simulink model "DDPGImpedance"  (R2024b)
settings: Solver=ode4  StartTime=0.001  StopTime=28  FixedStep=1e-4  RelTol=1e-3
libraries: simulink x2, slpidlib x1, rllib x1
settings Model: PacingRate=2  Creator=edwar  LastModifiedBy=edwar

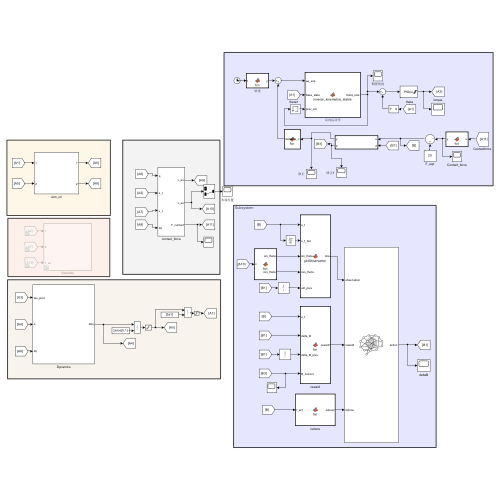
[thumbnail: Simulink's stored preview of the top-level diagram]
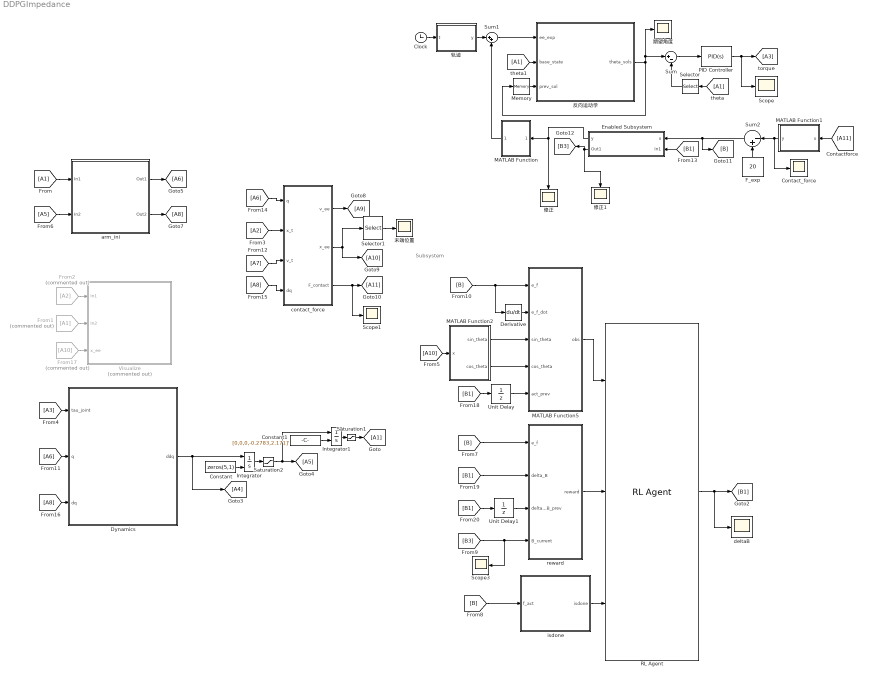
== system DDPGImpedance ==
  note: Subsystem
  Clock : Clock
  Constant : Constant  Value=zeros(5,1)
  Constant1 : Constant  Value=[0,0,0,-0.2783,2.171]'
  Contact_force : Scope
  Derivative : Derivative
  Dynamics : Subsystem
  Enabled Subsystem : Subsystem  TreatAsAtomicUnit=on
  F_exp : Constant  Value=20
  From1 : From  Commented=on  GotoTag=A1
  From17 : From  Commented=on  GotoTag=A10
  From2 : From  Commented=on  GotoTag=A2
  Integrator : Integrator  InitialConditionSource=external  InitialCondition=[0,0,0,0,0]'
  Integrator1 : Integrator  InitialConditionSource=external  InitialCondition=zeros(5,1)
  MATLAB Function : MATLAB Function  TreatAsAtomicUnit=on
  MATLAB Function1 : MATLAB Function  TreatAsAtomicUnit=on
  MATLAB Function2 : MATLAB Function  TreatAsAtomicUnit=on
  MATLAB Function5 : MATLAB Function  TreatAsAtomicUnit=on
  Memory : Memory  InitialCondition=[0;0]  InheritSampleTime=on
  PID Controller : slpidlib/PID Controller  Controller=PID  Form=Parallel  TimeDomain=Continuous-time  UseExternalTs=off  SampleTime=-1  IntegratorMethod=Forward Euler  FilterMethod=Forward Euler  ControllerParametersSource=internal  P=0.5  I=0  UseKiTs=off  D=0.8  UseExternalDerivativeSource=off  N=100  UseFilter=on  TunerSelectOption=Transfer Function Based (PID Tuner App)  InitialConditionSource=internal  InitialConditionForIntegrator=0  InitialConditionForFilter=0  DifferentiatorICPrevScaledInput=0  ExternalReset=none  TrackingMode=off  Kt=1  LimitOutput=on  SatLimitsSource=internal  UpperSaturationLimit=1.4  LowerSaturationLimit=-1.4  LinearizeAsGain=on  AntiWindupMode=none  Kb=1  LimitIntegrator=off  UpperIntegratorSaturationLimit=inf  LowerIntegratorSaturationLimit=-inf  POutMin=[]  POutMax=[]  IOutMin=[]  IOutMax=[]  DOutMin=[]  DOutMax=[]  NOutMin=[]  NOutMax=[]  SumOutMin=[]  SumOutMax=[]  SaturationOutMin=[]  SaturationOutMax=[]  PParamMin=[]  PParamMax=[]  IParamMin=[]  IParamMax=[]  DParamMin=[]  DParamMax=[]  NParamMin=[]  NParamMax=[]  KbParamMin=[]  KbParamMax=[]  KtParamMin=[]  KtParamMax=[]  KbOutMin=[]  KbOutMax=[]  KtOutMin=[]  KtOutMax=[]  IntegratorOutMin=[]  IntegratorOutMax=[]  FilterOutMin=[]  FilterOutMax=[]  SumI1OutMin=[]  SumI1OutMax=[]  SumI2OutMin=[]  SumI2OutMax=[]  SumI3OutMin=[]  SumI3OutMax=[]  SumI4OutMin=[]  SumI4OutMax=[]  SumDOutMin=[]  SumDOutMax=[]  DifferentiatorOutMin=[]  DifferentiatorOutMax=[]  FilterDiffOutCoefMin=[]  FilterDiffOutCoefMax=[]  ReciprocalOutMin=[]  ReciprocalOutMax=[]  SumDenOutMin=[]  SumDenOutMax=[]  SumNumOutMin=[]  SumNumOutMax=[]  DivideOutMin=[]  DivideOutMax=[]  UdiffTsProdOutMin=[]  UdiffTsProdOutMax=[]  NTsProdOutMin=[]  NTsProdOutMax=[]  UintegralTsProdOutMin=[]  UintegralTsProdOutMax=[]  UngainTsProdOutMin=[]  UngainTsProdOutMax=[]  ClampingZeroOutDataTypeStr=Inherit: Inherit via back propagation  ClampingZeroOutMin=[]  ClampingZeroOutMax=[]  FilterDenConstantOutDataTypeStr=Inherit: Inherit via back propagation  FilterDenConstantOutMin=[]  FilterDenConstantOutMax=[]  PCopyOutDataTypeStr=Inherit: Inherit via back propagation  PCopyOutMin=[]  PCopyOutMax=[]  NCopyOutDataTypeStr=Inherit: Inherit via back propagation  NCopyOutMin=[]  NCopyOutMax=[]  IntegratorContinuousStateAttributes=''  IntegratorStateMustResolveToSignalObject=off  IntegratorRTWStateStorageClass=Auto  FilterContinuousStateAttributes=''  FilterStateMustResolveToSignalObject=off  FilterRTWStateStorageClass=Auto  ParallelPVariant=InternalParameters  IdealPVariant=Disabled  IVariant=InternalParameters  DVariant=InternalParameters  IntegratorVariant=Continuous  SatVariant=Enabled  AWVariant=Passthrough  PCopyVariant=Disabled  TRVariant=Disabled  FdbkBlocksVariant=Forward  IdealPFdbkVariant=Disabled  SatFdbkVariant=Disabled  DerivativeFilterVariant=ContFilter  NVariant=InternalParameters  NCopyVariant=Disabled  FilterICVariant=InternalICsFilter  IntegratorICVariant=InternalICs  ExternalResetVariant=Disabled  TRSumVariant=Passthrough  SumFdbkVariant=Disabled  SumVariant=Sum_PID  TsampFilterVariant=InternalTs  TsampNgainVariant=Passthrough  TsampIntegralVariant=Disabled_SignalSpec  ExternalSaturationOutDataTypeStr=Inherit: Same as second input  DerivativeSourceVariant=ErrorSignal  PreIntVariant=InternalPreInt
  RL Agent : rllib/RL Agent  Agent=agent  ExternalActionAsInput=off  ProvideLastAction=off  ProvideCumRwd=off  TreatAsDirectFeedthrough=on  UseStrictObservationDataTypes=off
  Saturation1 : Saturate  UpperLimit=[1.5,1.5,5*pi,2.5,2.5]'  LowerLimit=[-1.5,-1.5,-5*pi,-2.5,-2.5]'
  Saturation2 : Saturate  UpperLimit=[0.075,0.075,pi/6,4.2,4.2]'  LowerLimit=[-0.075,-0.075,-pi/6,-4.2,-4.2]'
  Scope : Scope
  Scope1 : Scope
  Scope3 : Scope
  Selector : Selector  InputPortWidth=5  IndexOptions=Index vector (dialog)  Indices=[4 5]  OutputSizes=1
  Selector1 : Selector  InputPortWidth=2  IndexOptions=Index vector (dialog)  Indices=[2]  OutputSizes=1
  Sum : Sum  Inputs=|+-
  Sum1 : Sum  Inputs=|++
  Sum2 : Sum  Inputs=|-+
  Unit Delay : UnitDelay  SampleTime=-1  HasFrameUpgradeWarning=on
  Unit Delay1 : UnitDelay  SampleTime=-1  HasFrameUpgradeWarning=on
  Visualize : Subsystem  Commented=on
  arm_ini : Subsystem
  contact_force : Subsystem
  deltaB : Scope
  isdone : MATLAB Function  TreatAsAtomicUnit=on
  reward : MATLAB Function  TreatAsAtomicUnit=on
  修正 : Scope
  修正1 : Scope
  反向运动学 : MATLAB Function  TreatAsAtomicUnit=on
  期望角度 : Scope
  末端位置 : Scope
  轨迹 : MATLAB Function  TreatAsAtomicUnit=on
  wires:
  Enabled Subsystem/1(y) -> 修正/1, MATLAB Function/1(delta_n)
  Integrator/1 -> Saturation2/1
  contact_force/1(v_ee) -> [A9]
  Dynamics/1(ddq) -> [A4], Integrator/1
  Sum1/1 -> 反向运动学/1(ee_exp)
  Sum/1 -> PID Controller/1
  [A7] -> contact_force/3(v_t)
  [A8] -> Dynamics/3(dq)
  [A5] -> arm_ini/2(In2)
  Memory/1 -> 反向运动学/3(prev_sol)
  MATLAB Function/1(dxdy) -> Sum1/2
  arm_ini/2(Out2) -> [A8]
  [A1] -> 反向运动学/2(base_state)
  From2/1 -> Visualize/1(In1)
  [A6] -> contact_force/1(q)
  轨迹/1(y) -> Sum1/1
  Saturation2/1 -> Integrator1/1, [A5]
  MATLAB Function1/1(y) -> Sum2/1, Contact_force/1
  [A1] -> arm_ini/1(In1)
  contact_force/2(x_ee) -> Selector1/1, [A10]
  PID Controller/1 -> Scope/1, [A3]
  [A2] -> contact_force/2(x_t)
  From1/1 -> Visualize/2(In2)
  Constant1/1 -> Integrator1/2
  Selector/1 -> Sum/2
  Constant/1 -> Integrator/2
  [A11] -> MATLAB Function1/1(u)
  反向运动学/1(theta_sols) -> 期望角度/1, Sum/1, Memory/1
  [A6] -> Dynamics/2(q)
  F_exp/1 -> Sum2/2
  [A1] -> Selector/1
  Integrator1/1 -> Saturation1/1
  Saturation1/1 -> [A1]
  Clock/1 -> 轨迹/1(t)
  [A3] -> Dynamics/1(tau_joint)
  arm_ini/1(Out1) -> [A6]
  [A8] -> contact_force/4(dq)
  contact_force/3(F_contact) -> Scope1/1, [A11]
  Sum2/1 -> Enabled Subsystem/1(u), [B]
  [B1] -> Enabled Subsystem/2(In1)
  Enabled Subsystem/2(Out1) -> 修正1/1, [B3]
  From17/1 -> Visualize/3(x_ee)
  [B1] -> Unit Delay/1
  [B1] -> Unit Delay1/1
  [B1] -> reward/2(delta_B)
  MATLAB Function2/2(cos_theta) -> MATLAB Function5/4(cos_theta)
  Unit Delay1/1 -> reward/3(delta_B_prev)
  reward/1(reward) -> RL Agent/2
  isdone/1(isdone) -> RL Agent/3
  [B] -> reward/1(e_f)
  MATLAB Function5/1(obs) -> RL Agent/1
  [B3] -> reward/4(B_current), Scope3/1
  Derivative/1 -> MATLAB Function5/2(e_f_dot)
  [B] -> isdone/1(f_act)
  Unit Delay/1 -> MATLAB Function5/5(act_prev)
  [A10] -> MATLAB Function2/1(x)
  RL Agent/1 -> [B1], deltaB/1
  MATLAB Function2/1(sin_theta) -> MATLAB Function5/3(sin_theta)
  [B] -> MATLAB Function5/1(e_f), Derivative/1
  Selector1/1 -> 末端位置/1

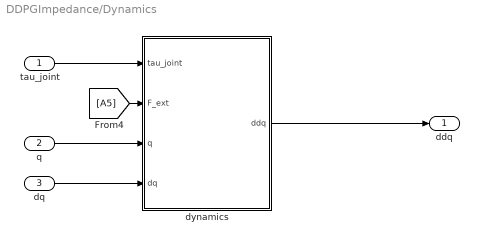
== system DDPGImpedance/Dynamics ==
  tau_joint : Inport
  q : Inport  Port=2
  dq : Inport  Port=3
  dynamics : MATLAB Function  TreatAsAtomicUnit=on
  ddq : Outport
  wires:
  tau_joint/1 -> dynamics/1(tau_joint)
  [A5] -> dynamics/2(F_ext)
  dq/1 -> dynamics/4(dq)
  dynamics/1(ddq) -> ddq/1
  q/1 -> dynamics/3(q)

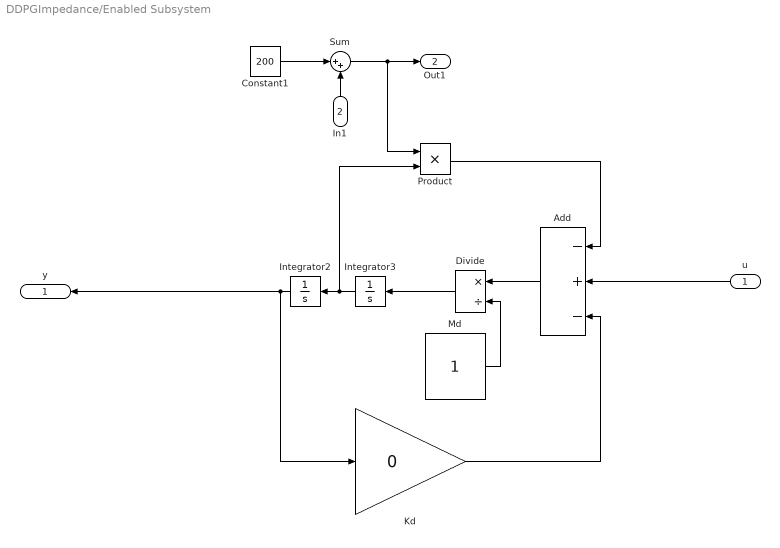
== system DDPGImpedance/Enabled Subsystem ==
  u : Inport
  In1 : Inport  Port=2
  Add : Sum  Inputs=-+-
  Constant1 : Constant  Value=200
  Divide : Product  Inputs=*/
  Integrator2 : Integrator
  Integrator3 : Integrator
  Kd : Gain  Gain=0
  Md : Constant
  Product : Product
  Sum : Sum  Inputs=|++
  y : Outport
  Out1 : Outport  Port=2
  wires:
  Md/1 -> Divide/2
  Product/1 -> Add/1
  Kd/1 -> Add/3
  Add/1 -> Divide/1
  u/1 -> Add/2
  Integrator2/1 -> y/1, Kd/1
  Divide/1 -> Integrator3/1
  Integrator3/1 -> Product/2, Integrator2/1
  Constant1/1 -> Sum/1
  Sum/1 -> Out1/1, Product/1
  In1/1 -> Sum/2

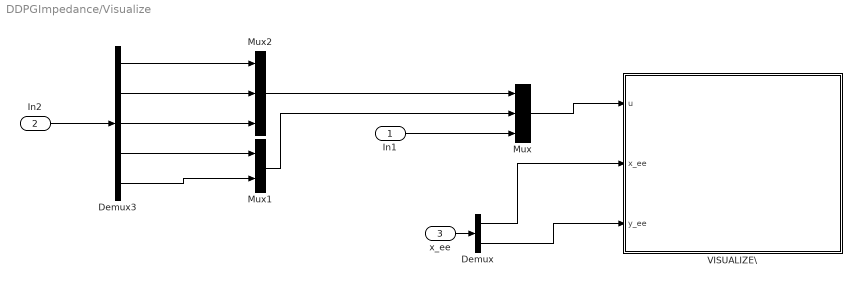
== system DDPGImpedance/Visualize ==
  In1 : Inport
  In2 : Inport  Port=2
  x_ee : Inport  Port=3
  Demux : Demux  Outputs=2
  Demux3 : Demux  Outputs=5
  Mux : Mux  Inputs=3
  Mux1 : Mux  Inputs=2
  Mux2 : Mux  Inputs=3
  VISUALIZE\ : MATLAB Function  TreatAsAtomicUnit=on
  wires:
  Demux3/4 -> Mux1/1
  Mux/1 -> VISUALIZE\/1(u)
  Demux3/3 -> Mux2/3
  Mux2/1 -> Mux/1
  Demux3/2 -> Mux2/2
  Mux1/1 -> Mux/2
  Demux3/5 -> Mux1/2
  Demux3/1 -> Mux2/1
  In1/1 -> Mux/3
  In2/1 -> Demux3/1
  x_ee/1 -> Demux/1
  Demux/2 -> VISUALIZE\/3(y_ee)
  Demux/1 -> VISUALIZE\/2(x_ee)

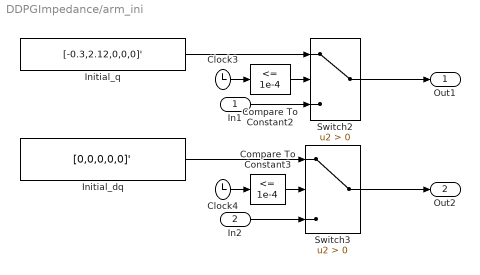
== system DDPGImpedance/arm_ini ==
  In1 : Inport
  In2 : Inport  Port=2
  Clock3 : Clock
  Clock4 : Clock
  Compare To Constant2 : simulink/Logic and Bit Operations/Compare To Constant  relop=<=  const=1e-4  OutDataTypeStr=boolean
  Compare To Constant3 : simulink/Logic and Bit Operations/Compare To Constant  relop=<=  const=1e-4  OutDataTypeStr=boolean
  Initial_dq : Constant  Value=[0,0,0,0,0]'
  Initial_q : Constant  Value=[-0.3,2.12,0,0,0]'
  Switch2 : Switch  Criteria=u2 > Threshold  SaturateOnIntegerOverflow=off  InputSameDT=off
  Switch3 : Switch  Criteria=u2 > Threshold  SaturateOnIntegerOverflow=off  InputSameDT=off
  Out1 : Outport
  Out2 : Outport  Port=2
  wires:
  In1/1 -> Switch2/3
  Compare To Constant3/1 -> Switch3/2
  Switch3/1 -> Out2/1
  Initial_dq/1 -> Switch3/1
  Clock3/1 -> Compare To Constant2/1
  In2/1 -> Switch3/3
  Clock4/1 -> Compare To Constant3/1
  Initial_q/1 -> Switch2/1
  Compare To Constant2/1 -> Switch2/2
  Switch2/1 -> Out1/1

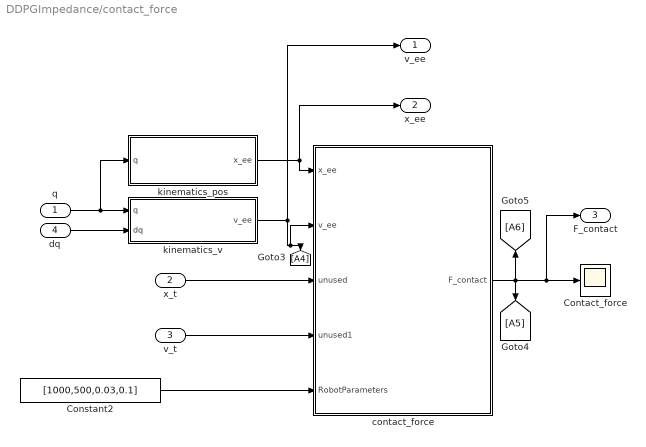
== system DDPGImpedance/contact_force ==
  q : Inport
  x_t : Inport  Port=2
  v_t : Inport  Port=3
  dq : Inport  Port=4
  Constant2 : Constant  Value=[1000,500,0.03,0.1]
  Contact_force : Scope
  contact_force : MATLAB Function  TreatAsAtomicUnit=on  SystemSampleTime=0.01
  kinematics_pos : MATLAB Function  TreatAsAtomicUnit=on
  kinematics_v : MATLAB Function  TreatAsAtomicUnit=on
  v_ee : Outport
  x_ee : Outport  Port=2
  F_contact : Outport  Port=3
  wires:
  kinematics_v/1(v_ee) -> v_ee/1, contact_force/2(v_ee), [A4]
  contact_force/1(F_contact) -> [A5], [A6], Contact_force/1, F_contact/1
  kinematics_pos/1(x_ee) -> x_ee/1, contact_force/1(x_ee)
  x_t/1 -> contact_force/3(unused)
  Constant2/1 -> contact_force/5(RobotParameters)
  q/1 -> kinematics_pos/1(q), kinematics_v/1(q)
  v_t/1 -> contact_force/4(unused1)
  dq/1 -> kinematics_v/2(dq)

== matlab function DDPGImpedance/reward ==
  data: e_f input; delta_B input; delta_B_prev input; reward output; B_current input
function reward = fcn(e_f, delta_B, delta_B_prev, B_current)     
                                                                %#codegen                                                        
                                                                %#ok<INUSD>                                                      
                                                                wForce = 0.5;                                                    
                                                                wSmooth = 0.01;                                                  
                                                                actionLimit = 100.0;                                             
                                                                
                                                                forceReward = exp(-0.01 * e_f^2);                                
                                                                normalizedActionRate = (delta_B - delta_B_prev) / actionLimit;   
                                                                reward = wForce * forceReward - wSmooth * normalizedActionRate^2;
                                                                
                                                                if abs(e_f) > 20.0                                               
                                                                    reward = reward - 0.01 * exp(0.3 * (abs(e_f) - 20.0));       
                                                                end                                                              
                                                                end

== matlab function DDPGImpedance/反向运动学 ==
  data: ee_exp input; theta_sols output; base_state input; prev_sol input
function theta_sols = inverse_kinematics_stable(ee_exp, base_state, prev_sol)
    %#codegen
    b_b = 0.151; L1 = 0.225; L2 = 0.276;
    
    x_t = ee_exp(1); y_t = ee_exp(2);
    x_b = base_state(1); y_b = base_state(2); theta_b = base_state(3);
    
    % 当前关节角（带保护）
    if length(base_state) >= 5
        q_current = [base_state(4); base_state(5)];
    else
        q_current = [0; 0];
    end
    
    % 使用上一次成功解作为参考，确保是列向量
    if nargin < 3 || isempty(prev_sol)
        ref = q_current(:);  % 确保是列向量
    else
        ref = prev_sol(:);   % 确保是列向量
    end
   
    
    % 坐标变换
    dx = x_t - x_b; dy = y_t - y_b;
    x_prime = cos(theta_b)*dx + sin(theta_b)*dy - b_b;
    y_prime = -sin(theta_b)*dx + cos(theta_b)*dy;
    
    r_sq = x_prime^2 + y_prime^2;
    r = sqrt(r_sq);
    
    % 可达性检查
    if r > (L1 + L2) || r < abs(L1 - L2) || r < 1e-6
        theta_sols = ref(:);  % 确保输出是列向量
        return;
    end
    
    cos_theta2 = (r_sq - L1^2 - L2^2) / (2 * L1 * L2);
    cos_theta2 = max(-1.0, min(1.0, cos_theta2));
    
    sin_theta2 = sqrt(1 - cos_theta2^2);   % 正值
    
    angle_base = atan2(y_prime, x_prime);
    
    % 两组解（确保都是列向量）
    theta2_a = atan2( sin_theta2, cos_theta2);
    theta2_b = atan2(-sin_theta2, cos_theta2);
    
    theta1_a = angle_base - atan2(L2*sin_theta2, L1 + L2*cos_theta2);
    theta1_b = angle_base - atan2(-L2*sin_theta2, L1 + L2*cos_theta2);
    
    sol_a = [theta1_a; theta2_a];
    sol_b = [theta1_b; theta2_b];
    
    % ================== 关键改进：连续性处理 ==================
    % 1. 先把两组解都缠绕到最接近参考解
    sol_a = ref + wrapToPi(sol_a - ref);
    sol_b = ref + wrapToPi(sol_b - ref);
    
    % 2. 计算代价（距离 + 配置切换惩罚）
    % 现在ref(1)和ref(2)都可以安全访问
    cost_a = sum((sol_a - ref).^2) + 0.5 * abs(sol_a(2) - ref(2));
    cost_b = sum((sol_b - ref).^2) + 0.5 * abs(sol_b(2) - ref(2));  
    % 3. 优先选择最接近的
    if cost_a <= cost_b
        theta_sols = sol_a;
    else
        theta_sols = sol_b;
    end
    
    % 最终再对当前状态做一次小调整（防止累计漂移）
    theta_sols = ref + wrapToPi(theta_sols - ref);
    theta_sols = theta_sols(:);  % 确保输出是列向量
end

== matlab function DDPGImpedance/轨迹 ==
  data: t input; y output
function y = fcn(t)
    A = 0.05;   % 振幅
    w = 2*pi/0.3; % 空间频率
    v = 0.01;   % x方向运动速度
    y0 = 0.2;  % 基准高度
    x_start = 0.28;
    x_stop  = 0.58;

    % 计算不受限制的 x 位置
    x = x_start + v * t;
    
    % 限制在 0.65
    if x > x_stop
        x = x_stop;
    end
    
    y = zeros(2,1);
    y(1) = x;
    y(2) = 0.2;
end

== matlab function DDPGImpedance/MATLAB Function2 ==
  data: x input; sin_theta output; cos_theta output
function [sin_theta,cos_theta] = fcn(x)
w = 2*pi/0.3;
x_start = 0.28;
x = x(1);
theta = w * (x - x_start);

% 2. 计算正交相位信号
sin_theta = sin(theta);
cos_theta = cos(theta);

== matlab function DDPGImpedance/Dynamics/dynamics ==
  data: tau_joint input; F_ext input size=[2,1]; q input size=[5,1]; ddq output size=[5,1]; dq input size=[5,1]
function ddq  = robot_dynamics(tau_joint, F_ext, q, dq)
    % 平面二连杆机器人动力学模型
    % 输入: tau_joint (2x1), F_ext (2x1?), q (5x1), dq (5x1?)
    % 输出: ddq (5x1)


    % 构建力矩向量（5维，前三个分量为0，假设前3是基座自由度不受控）
    tau_control = zeros(5,1);
    tau_control(4:5) = tau_joint(:);  % 关节控制力矩

    J = jacobian_matrix(q);

    % 接触力映射到关节空间
    if ~isempty(F_ext)
        tau_contact = -J' * F_ext(:);
    else
        tau_contact = zeros(5,1);
    end

    tau_total = tau_control + tau_contact;
    damping_coeff = 0.05;  % 0.02 ~ 0.1
    tau_damping = -damping_coeff * dq;  % 5x1，对所有自由度加线性阻尼
    tau_total = tau_total + tau_damping;
    [D, C] = dynamics_model(q, dq); 
    det_D = det(D);
    cond_D = cond(D);
    % 加速度
    ddq = D \ (tau_total - C);
end

== matlab function DDPGImpedance/MATLAB Function1 ==
  data: u input; y output
function y = fcn(u)
    y = abs(u(2));
end

== matlab function DDPGImpedance/contact_force/contact_force ==
  data: x_ee input; F_contact output double size=[2,1]; v_ee input; unused input; unused1 input; RobotParameters input
function F_contact = contact_force(x_ee, v_ee, ~, ~, RobotParameters)
    % 预分配接触力
    F_contact = zeros(2,1);   
    x_ee = x_ee(:);
    v_ee = v_ee(:);
    
    % 提取参数
    K    = RobotParameters(1);
    B    = RobotParameters(2);
    R_ee = RobotParameters(3); % 末端工具半径
    
    %% 正弦曲面参数 (固定墙体在上方，高度带有 0.2 偏移)
    A = 0.05;
    w = 2*pi/0.3;
    y0 = 0.2;
    x = x_ee(1);
    y = x_ee(2);
    
    %% 1. 计算当前 X 位置对应的曲面 Y 高度
    % 纯 Y 方向模型不需要计算导数 dydx 了
    y_surface = 0.2;
    
    %% 2. 计算纯 Y 方向的穿透深度
    % 机械臂在下方，最上沿的坐标是 y + R_ee
    % 当最上沿超过曲面高度时，发生接触
    penetration = (y + R_ee) - y_surface;
    
    if penetration > 0
        %% 3. 计算沿 Y 方向挤压墙体的速度
        % v_ee(2) 是末端在世界坐标系 Y 方向的速度
        % 因为墙在上方，向上运动（vy > 0）代表正在挤入墙体
        v_in = v_ee(2); 
        
        %% 4. 计算接触力的大小
        F_spring = K * penetration;
        F_damp   = B * max(v_in, 0); % 只有向上挤压墙体时才产生阻尼力
        
        %% 5. 输出接触力向量（方向绝对沿世界坐标 Y 轴向下）
        % 墙体在上方，给机械臂的弹力与阻尼力必然是垂直向下的
        F_contact(1) = 0;                  % X 方向不受力
        F_contact(2) = -(F_spring + F_damp); % Y 方向受力向下
    end
end

== matlab function DDPGImpedance/Visualize/VISUALIZE\ ==
  settings: updateMethod=DISCRETE
  data: u input; x_ee input; y_ee input
function visualize_arm(u,x_ee,y_ee)

% ================================================
% 平面二连杆自由基座机械臂 + 水平墙面 可视化（Simulink专用）
% 输入 u = [x_b, y_b, theta_b, q1, q2, x_ee, y_ee]
%       前5个：用于绘制机械臂本体
%       后2个：直接传入的末端执行器位置，用于绘制轨迹
% ================================================

% ================== 参数（直接使用您提供的值） ==================
b_b   = 0.151;   % 基座质心到关节1距离 (m)
l1    = 0.225;   % 连杆1长度 (m)
l2    = 0.276;   % 连杆2长度 (m)
R_ee  = 0.03;    % 末端执行器半径 (m)

% ================== 持久化图形对象（只创建一次） ==================
persistent h_fig h_base h_link1 h_link2 h_ee h_surface ...
           ee_offset_x ee_offset_y base_vertices
persistent call_counter visualize_every
persistent h_traj traj_x traj_y max_traj_points traj_idx  % 轨迹相关

if isempty(call_counter)
    call_counter = 0;
    visualize_every = 50;
end

call_counter = call_counter + 1;
if mod(call_counter, visualize_every) ~= 0
    return;
end

if isempty(h_fig)
    h_fig = figure();
    ax = gca;
    hold(ax, 'on');
    grid(ax, 'on');
    axis(ax, 'equal');
    xlim(ax, [-0.5 1]);
    ylim(ax, [-0.5 1]);
    xlabel(ax, 'X (m)');
    ylabel(ax, 'Y (m)');
    
    % 初始化基座线段
    base_size = 0.4;           
    half = base_size / 2;
    base_vertices = [ ...
        -half, -half;
         half, -half;
         half,  half;
        -half,  half;
        -half, -half];
    
    % 创建基座
    h_base = patch(ax, ...
        'XData', base_vertices(:,1), 'YData', base_vertices(:,2), ...
        'FaceColor', 'k', ...     
        'EdgeColor', [0.5 0.5 0.5], ...            
        'LineWidth', 2.5, ...
        'FaceAlpha', 0.85, ...               
        'DisplayName', 'Base');
        
    h_link1 = line(ax, [0 0], [0 0], 'Color', [0.5 0.5 0.5], 'LineWidth', 4, 'DisplayName', 'L1');
    h_link2 = line(ax, [0 0], [0 0], 'Color', [0.5 0.5 0.5], 'LineWidth', 4, 'DisplayName', 'L2');
    
    % 末端执行器圆圈
    theta_c = linspace(0, 2*pi, 50);
    ee_offset_x = R_ee * cos(theta_c);
    ee_offset_y = R_ee * sin(theta_c);
    h_ee = line(ax, ee_offset_x, ee_offset_y, ...
                'Color', 'b', 'LineWidth', 1.5, 'DisplayName', 'End');
               
    % 物体表面（波浪形）
    A  = 0.05;          
    w  = 2*pi/0.3;      
    y0 = 0.2;          
    x_surface = linspace(-0.5, 1, 500);
    y_surface = A*sin(w*x_surface) + y0;
    h_surface = line(ax, x_surface, y_surface, ...
                     'Color', 'r', ...
                     'LineWidth', 2, ...
                     'DisplayName', 'Object');
    
    % 【新增】初始化轨迹线
    h_traj = line(ax, nan, nan, ...
                  'Color', [0 0.5 0], ...      % 深绿色
                  'LineWidth', 1.5, ...
                  'LineStyle', '-', ...
                  'DisplayName', 'EE Trajectory');
    
    % 【新增】初始化轨迹存储
    max_traj_points = 100000;
    traj_x = nan(max_traj_points, 1);
    traj_y = nan(max_traj_points, 1);
    traj_idx = 1;
    
    legend(ax, 'Location', 'northwest');
end

% ================== 提取输入 ==================
xb     = u(1);
yb     = u(2);
thetab = u(3);
q1     = u(4);
q2     = u(5);


% ================== 正运动学（用于绘制连杆，不含末端） ==================
x_j1 = xb + b_b * cos(thetab);
y_j1 = yb + b_b * sin(thetab);
x_j2 = x_j1 + l1 * cos(thetab + q1);
y_j2 = y_j1 + l1 * sin(thetab + q1);
% 注意：这里不再计算 x_ee, y_ee，而是直接使用传入的

% ================== 更新轨迹（使用传入的末端位置） ==================
traj_x(traj_idx) = x_ee;
traj_y(traj_idx) = y_ee;

traj_idx = traj_idx + 1;
if traj_idx > max_traj_points
    traj_idx = 1;
end

% 获取有效轨迹数据
if traj_idx > 1
    valid_x = traj_x(1:traj_idx-1);
    valid_y = traj_y(1:traj_idx-1);
else
    valid_x = traj_x;
    valid_y = traj_y;
end
set(h_traj, 'XData', valid_x, 'YData', valid_y);

% ================== 更新图形 ==================
R = [cos(thetab), -sin(thetab); 
     sin(thetab),  cos(thetab)];
 
rotated = (R * base_vertices')';          
abs_x = xb + rotated(:,1);
abs_y = yb + rotated(:,2);

set(h_base, 'XData', abs_x, 'YData', abs_y);
set(h_link1, 'XData', [x_j1, x_j2], 'YData', [y_j1, y_j2]);
set(h_link2, 'XData', [x_j2, x_ee], 'YData', [y_j2, y_ee]);  % 使用传入的末端位置
set(h_ee,    'XData', x_ee + ee_offset_x, 'YData', y_ee + ee_offset_y);  % 使用传入的末端位置

drawnow limitrate;

end

== matlab function DDPGImpedance/contact_force/kinematics_pos ==
  data: x_ee output; q input
function x_ee  = forward_kinematics(q)
    x_ee = zeros(1,2);
    % q = [x_b; y_b; theta_b; theta1; theta2]
    x_b = q(1); y_b = q(2); theta_b = q(3);
    theta1 = q(4); theta2 = q(5);
    b_b = 0.151;
    L1 = 0.225; L2 = 0.276;  % 连杆长度
    
    % 相对基座的末端位置
    x_rel = b_b + L1*cos(theta1) + L2*cos(theta1+theta2);
    y_rel = L1*sin(theta1) + L2*sin(theta1+theta2);
    
    % 转换到世界坐标系
    R = [cos(theta_b) -sin(theta_b); sin(theta_b) cos(theta_b)];
    pos_world = R * [x_rel; y_rel] + [x_b; y_b];
    
    x_ee(1) = pos_world(1);
    x_ee(2) = pos_world(2);
end

== matlab function DDPGImpedance/MATLAB Function ==
  data: delta_n input; dxdy output
function dxdy = fcn(delta_n)
    dxdy = zeros(2, 1);
%#codegen

    % X 方向不作任何阻抗修正，防止前进方向死锁
    dxdy(1) = 0; 
    
    % Y 方向直接赋修正量
    % 注：如果你的 delta_n 物理意义是指向“上方”为正，而你想让它往下压，这里可以加负号（-delta_n）
    dxdy(2) = delta_n; 
    
end

== matlab function DDPGImpedance/MATLAB Function5 ==
  data: e_f input; e_f_dot input; sin_theta input; cos_theta input; obs output; act_prev input
function obs = getObservation(e_f, e_f_dot, sin_theta, cos_theta, act_prev)     
                                                                               %#codegen                                                                       
                                                                               F_MAX = 30.0;                                                                   
                                                                               FD_MAX = 200.0;                                                                 
                                                                               ACT_MAX = 100.0;                                                                
                                                                               
                                                                               obs = [e_f / F_MAX; e_f_dot / FD_MAX; sin_theta; cos_theta; act_prev / ACT_MAX];
                                                                               obs = min(max(obs, -1.0), 1.0);                                                 
                                                                               end

== matlab function DDPGImpedance/contact_force/kinematics_v ==
  data: q input; v_ee output; dq input
function v_ee = forward_kinematics_v(q,dq)
J = jacobian_matrix(q);
% 计算末端速度
v_ee = (J * dq)';
end

== matlab function DDPGImpedance/isdone ==
  data: isdone output double size=1; f_act input double
function isdone = fcn(f_act)
%#codegen
% 该函数用于判断安全边界，输出布尔值控制仿真重置

    fail_force = abs(f_act) >30.0;     % 设定力保护上限 30



    isdone =(fail_force);
    isdone = double(real(isdone));
end
